simulink model "VOO"  (R2022b)
settings: Solver=FixedStepAuto  StartTime=0.0  StopTime=10.0  FixedStep=1e-3  RelTol=1e-3  EnableMultiTasking=on
undefined symbols (not defined in the file): D10, D11, D12, D2, D4, D5, D7, D8, D9, PTA0, PTA2, PTB23, PTB9, PTC3, PTC4, PTD0, PTD2, PTD3
libraries: frdmk64flib x9
settings Model: ExtModeTrigDuration=5  Creator=clara  LastModifiedBy=pragy
settings OptimizationCC: EnhancedBackFolding=on  PassReuseOutputArgsAs=Individual arguments  ZeroExternalMemoryAtStartup=off  ZeroInternalMemoryAtStartup=off  MaxStackSize=64  OptimizeBlockOrder=speed  DifferentSizesBufferReuse=on  OptimizationCustomize=off  EfficientTunableParamExpr=on
settings DebuggingCC: ParameterTunabilityLossMsg=error
settings HardwareCC: ProdBitPerPointer=32  ProdBitPerSizeT=32  ProdBitPerPtrDiffT=32  ProdLargestAtomicInteger=Long  ProdLargestAtomicFloat=Double  ProdWordSize=32  ProdHWDeviceType=ARM Compatible->ARM Cortex
settings ModelReferenceCC: EnableRefExpFcnMdlSchedulingChecks=on
settings SFSimCC: MATLABDynamicMemAlloc=off
settings RTWCC: Description=Embedded Coder  SystemTargetFile=ert.tlc  HardwareBoard=NXP FRDM-K64F  TLCOptions="-aInlineSetEventsForThisBaseRateFcn=TLC_FALSE -aSuppressMultiTaskScheduler=TLC_FALSE  -aRateBasedStepFcn=0"  TemplateMakefile=ert_default_tmf  Toolchain=GNU Tools for ARM Embedded Processors
settings CodeAppCC: ForceParamTrailComments=on  IgnoreCustomStorageClasses=off  OperatorAnnotations=on  SimulinkDataObjDesc=on  SFDataObjDesc=on  InsertBlockDesc=on
settings ERTTargetCC: ExtModeTransport=4  ExtModeMexFile=sendToCommService

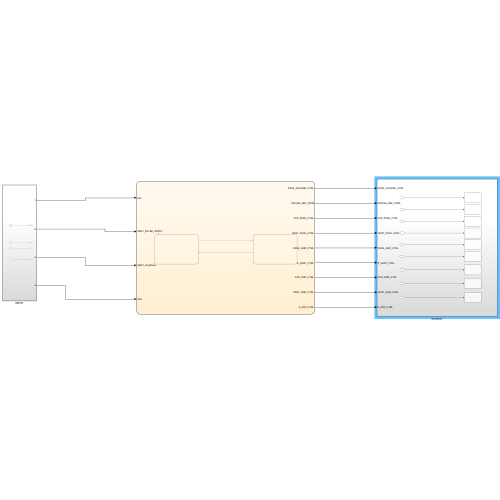
[thumbnail: Simulink's stored preview of the top-level diagram]
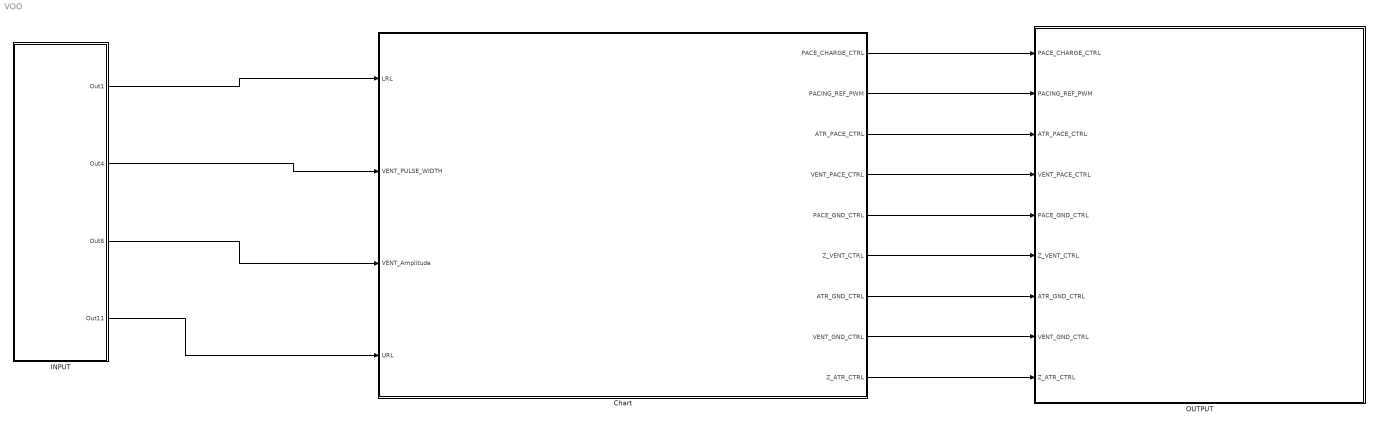
== system VOO ==
  Chart : Stateflow chart  TreatAsAtomicUnit=on
  "INPUT " : Subsystem
  OUTPUT : Subsystem
  wires:
  Chart/7(ATR_GND_CTRL) -> OUTPUT/7(ATR_GND_CTRL)
  Chart/3(ATR_PACE_CTRL) -> OUTPUT/3(ATR_PACE_CTRL)
  Chart/6(Z_VENT_CTRL) -> OUTPUT/6(Z_VENT_CTRL)
  Chart/8(VENT_GND_CTRL) -> OUTPUT/8(VENT_GND_CTRL)
  Chart/5(PACE_GND_CTRL) -> OUTPUT/5(PACE_GND_CTRL)
  Chart/9(Z_ATR_CTRL) -> OUTPUT/9(Z_ATR_CTRL)
  Chart/2(PACING_REF_PWM) -> OUTPUT/2(PACING_REF_PWM)
  "INPUT "/1(Out1) -> Chart/1(LRL)
  "INPUT "/3(Out6) -> Chart/3(VENT_Amplitude)
  Chart/1(PACE_CHARGE_CTRL) -> OUTPUT/1(PACE_CHARGE_CTRL)
  "INPUT "/2(Out4) -> Chart/2(VENT_PULSE_WIDTH)
  Chart/4(VENT_PACE_CTRL) -> OUTPUT/4(VENT_PACE_CTRL)
  "INPUT "/4(Out11) -> Chart/4(URL)

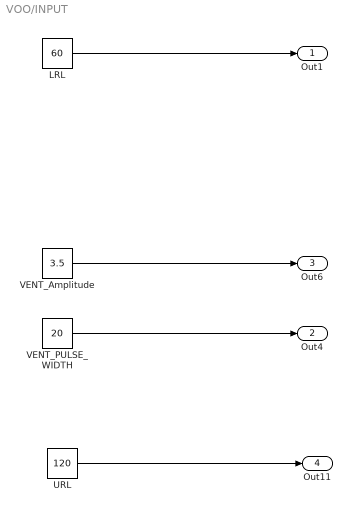
== system VOO/INPUT  ==
  LRL : Constant  Value=60
  URL : Constant  Value=120
  VENT_Amplitude : Constant  Value=3.5
  VENT_PULSE_WIDTH : Constant  Value=20
  Out1 : Outport
  Out4 : Outport  Port=2
  Out6 : Outport  Port=3
  Out11 : Outport  Port=4
  wires:
  LRL/1 -> Out1/1
  VENT_PULSE_WIDTH/1 -> Out4/1
  VENT_Amplitude/1 -> Out6/1
  URL/1 -> Out11/1

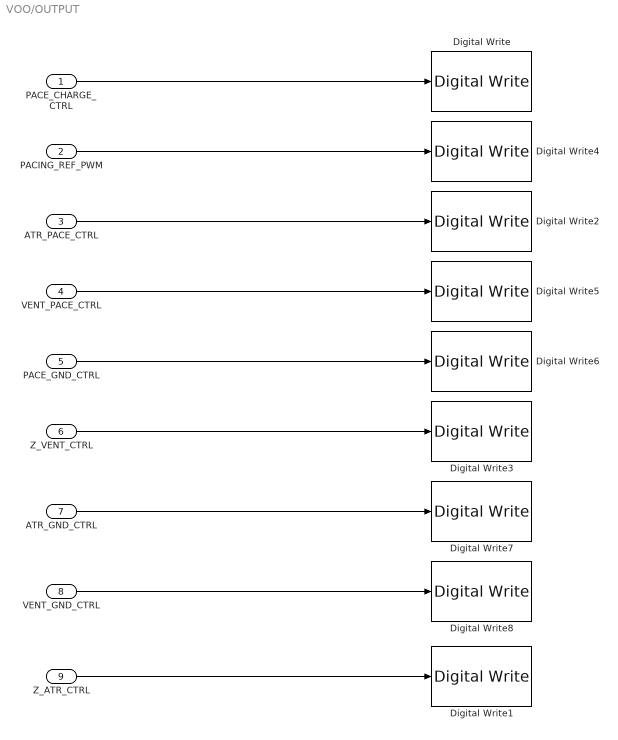
== system VOO/OUTPUT ==
  PACE_CHARGE_CTRL : Inport
  PACING_REF_PWM : Inport  Port=2
  ATR_PACE_CTRL : Inport  Port=3
  VENT_PACE_CTRL : Inport  Port=4
  PACE_GND_CTRL : Inport  Port=5
  Z_VENT_CTRL : Inport  Port=6
  ATR_GND_CTRL : Inport  Port=7
  VENT_GND_CTRL : Inport  Port=8
  Z_ATR_CTRL : Inport  Port=9
  Digital Write : frdmk64flib/Digital Write  Whichpin=PTB9 (D2)
  Digital Write1 : frdmk64flib/Digital Write  Whichpin=PTB23 (D4)
  Digital Write2 : frdmk64flib/Digital Write  Whichpin=PTA0 (D8)
  Digital Write3 : frdmk64flib/Digital Write  Whichpin=PTC3 (D7)
  Digital Write4 : frdmk64flib/Digital Write  Whichpin=PTA2 (D5)
  Digital Write5 : frdmk64flib/Digital Write  Whichpin=PTC4 (D9)
  Digital Write6 : frdmk64flib/Digital Write  Whichpin=PTD0 (D10)
  Digital Write7 : frdmk64flib/Digital Write  Whichpin=PTD2 (D11)
  Digital Write8 : frdmk64flib/Digital Write  Whichpin=PTD3 (D12)
  wires:
  PACE_CHARGE_CTRL/1 -> Digital Write/1
  PACING_REF_PWM/1 -> Digital Write4/1
  ATR_PACE_CTRL/1 -> Digital Write2/1
  VENT_PACE_CTRL/1 -> Digital Write5/1
  PACE_GND_CTRL/1 -> Digital Write6/1
  Z_VENT_CTRL/1 -> Digital Write3/1
  ATR_GND_CTRL/1 -> Digital Write7/1
  VENT_GND_CTRL/1 -> Digital Write8/1
  Z_ATR_CTRL/1 -> Digital Write1/1

== stateflow chart VOO/Chart ==
  state VOO
    entry:
    % charge condition for C22
    ATR_PACE_CTRL = false;
    VENT_PACE_CTRL = false;
    PACE_CHARGE_CTRL = true;
    % discharge condition for C21;
    VENT_GND_CTRL = true;
    PACE_GND_CTRL = true;
    ATR_GND_CTRL = false;
    Z_ATR_CTRL = false;
    Z_VENT_CTRL = false;
    %
    PACING_REF_PWM = 20*VENT_Amplitude;
  state Pacing_VOO
    entry:
    PACE_CHARGE_CTRL = false;
    PACE_GND_CTRL = true;
    ATR_PACE_CTRL = false;
    ATR_GND_CTRL = false;
    Z_ATR_CTRL = false;
    Z_VENT_CTRL = false;
    VENT_GND_CTRL = false;
    VENT_PACE_CTRL = true;
    %
  (default) -> VOO
  VOO -> Pacing_VOO : [after(60000/LRL - VENT_PULSE_WIDTH,msec)]
  Pacing_VOO -> VOO : [after(VENT_PULSE_WIDTH,msec)]
  data: PACE_CHARGE_CTRL output; PACING_REF_PWM output; ATR_PACE_CTRL output; VENT_PACE_CTRL output; PACE_GND_CTRL output; Z_VENT_CTRL output; ATR_GND_CTRL output; VENT_GND_CTRL output; Z_ATR_CTRL output; LRL input; VENT_PULSE_WIDTH input; VENT_Amplitude input; URL input
